simulink model "HQEV_MiL_20160830_integrate_r2017a"  (Simulink 8.9)
settings: Solver=FixedStepDiscrete  StartTime=0.0  StopTime=inf  FixedStep=0.01  RelTol=1e-3  EnableMultiTasking=on
PostLoadFcn:
  | , if any(exist('dsrtsu_mdlpostloadfcn', 'file') == [2, 3, 6]), try dsrtsu_mdlpostloadfcn('Execute', bdroot); catch fprintf('Error in PostLoadFcn (dsrtsu_mdlpostloadfcn) for model "%s":\n %s\n', bdroot, lasterr); end, end,
values from neighbouring files (symbols this model uses):
  Bat_C_Ah = 36    [parameter_V1.mat]
  Bat_ocv_xIndex = [5 10 20 30 40 50 60 70 80 90 95]    [parameter_V1.mat]
  Bat_ocv_z = [329 332 340 345 347 351 358 372 377 386 391]    [parameter_V1.mat]
  Bat_R_ohm_z = [4.41 3.46 1.57 1.07 0.76 0.63 0.55 0.44 0.41 0.4 0.4 3.14 ... (66 elements, 11x6)]    [parameter_V1.mat]
  Bat_SOC_Init = 90    [parameter_V1.mat]
  Env_hum_pct_Ambient = 30    [parameter_V1.mat]
  Env_Slope_deg = 0    [parameter_V1.mat]
  Env_Temp_degC_Ambient = 25    [parameter_V1.mat]
  Env_v_kmph_HWind = 0    [parameter_V1.mat]
  Reducer_F_i = 7.23    [parameter_V1.mat]
  Reducer_R_i = 7.23    [parameter_V1.mat]
  Veh =     [parameter_V1.mat]
  Veh_A_m2_Fr = 2.246    [parameter_V1.mat]
  Veh_F_Brake =     [parameter_V1.mat]
  Veh_fac_AirDrag = 0.326    [parameter_V1.mat]
  Veh_fac_WhDragFrict_0 = 0.011    [parameter_V1.mat]
  Veh_g_mps2_C = 9.81    [parameter_V1.mat]
  Veh_GainBrake =     [parameter_V1.mat]
  Veh_h_m_COGHigh = 0.5    [parameter_V1.mat]
  Veh_J_kgm2_Wh = 1.3635    [parameter_V1.mat]
  Veh_L_m_AxlBas = 2.63    [parameter_V1.mat]
  Veh_M_kg = 1427    [parameter_V1.mat]
  Veh_mu_Brake = 0.4    [parameter_V1.mat]
  Veh_mu_Tyre =     [parameter_V1.mat]
  Veh_num_FrictPair = 8    [parameter_V1.mat]
  Veh_pct_Brk = 70    [parameter_V1.mat]
  Veh_r_dyn =     [parameter_V1.mat]
  Veh_r_m_BrkDisk = 0.136    [parameter_V1.mat]
  Veh_rho_kgpm3_Air = 1.2258    [parameter_V1.mat]
undefined symbols (not defined in the file or in its folder): DiscIntNeverNeededParam, p_bool_False_M, p_bool_True_M
libraries: BaseOperationLib_Browser x38, simulink x8, DTQC_lib x1, ERR_lib x1, MQM_lib x1, PTCL_lib x1, PUD_lib x1, TQD_lib x1, TQR_lib x1, VMM_lib x1, ACCA_lib x1, BBCA_lib x1
(part 2 of 15)

== system HQEV_MiL_20160830_integrate_r2017a/MiL/Test_Integration/EGSM/EGSM ==
  In1 : Inport
  Bus Selector : BusSelector  OutputSignals=Drv.signal2.ParkButton (signal 11),Drv.signal2.SecurityButton (signal 12),Drv.signal2.EGSM_KnobPosition (signal 13),Drv.signal2.EGSM_ECOSButton (signal 14)
  Constant{,1..7} (8 alike) : Constant  Value=0
  Checksum_EGSM_1 : Outport
  EGSM_ParkButton : Outport  Port=2
  EGSM_SecurityButton : Outport  Port=3
  EGSM_KnobPosition : Outport  Port=4
  EGSMErrorStatus : Outport  Port=5
  EGSM_ECOSButton : Outport  Port=6
  LiveCounter_EGSM_1 : Outport  Port=7
  PowerSupplyStatus : Outport  Port=8
  EGSM_CANError : Outport  Port=9
  EGSM_LINError : Outport  Port=10
  EGSM_HallSensorError : Outport  Port=11
  EGSM_InternalError : Outport  Port=12
  wires:
  In1/1 -> Bus Selector/1
  Constant/1 -> Checksum_EGSM_1/1
  Constant1/1 -> EGSMErrorStatus/1
  Constant2/1 -> LiveCounter_EGSM_1/1
  Constant3/1 -> PowerSupplyStatus/1
  Constant4/1 -> EGSM_CANError/1
  Constant5/1 -> EGSM_LINError/1
  Constant6/1 -> EGSM_HallSensorError/1
  Constant7/1 -> EGSM_InternalError/1
  Bus Selector/1 -> EGSM_ParkButton/1  "<ParkButton (signal 11)>"
  Bus Selector/2 -> EGSM_SecurityButton/1  "<SecurityButton (signal 12)>"
  Bus Selector/3 -> EGSM_KnobPosition/1  "<EGSM_KnobPosition (signal 13)>"
  Bus Selector/4 -> EGSM_ECOSButton/1  "<EGSM_ECOSButton (signal 14)>"

== system HQEV_MiL_20160830_integrate_r2017a/MiL/Test_Integration/EPS/EPS ==
  Bus Creator : BusCreator  Inputs=2
  Subsystem2 : Subsystem
  EPS : Outport
  wires:
  Subsystem2/2(SteeringWheelAngleStatus) -> Bus Creator/2  "SteeringWheelAngleStatus"
  Subsystem2/1(EPSErrorStatus) -> Bus Creator/1  "EPSErrorStatus"
  Bus Creator/1 -> EPS/1

== system HQEV_MiL_20160830_integrate_r2017a/MiL/Test_Integration/ESP/Subsystem ==
  In1 : Inport
  ABS : Subsystem
  ASR : Subsystem
  ASR2 : Subsystem
  Bus Creator1 : BusCreator  Inputs=18
  Bus Creator2 : BusCreator  Inputs=6
  Bus Creator3 : BusCreator  Inputs=10
  Bus Creator4 : BusCreator  Inputs=4
  Bus Creator5 : BusCreator  Inputs=5
  Bus Creator6 : BusCreator  Inputs=6
  EPB : Subsystem
  YRS : Subsystem
  ESP : Outport
  wires:
  ABS/1(Checksum_ABS_1) -> Bus Creator1/1  "Checksum_ABS_1"
  ABS/2(WheelSpeed_FL) -> Bus Creator1/2  "WheelSpeed_FL"
  ABS/3(WheelSpeed_FR) -> Bus Creator1/3  "WheelSpeed_FR"
  ABS/4(ABS_VehicleSpeed) -> Bus Creator1/4  "ABS_VehicleSpeed"
  ABS/5(LiveCounter_ABS_1) -> Bus Creator1/5  "LiveCounter_ABS_1"
  ABS/6(Checksum_ABS_2) -> Bus Creator1/6  "Checksum_ABS_2"
  ABS/7(WheelSpeed_RL) -> Bus Creator1/7  "WheelSpeed_RL"
  ABS/8(WheelSpeed_RR) -> Bus Creator1/8  "WheelSpeed_RR"
  ABS/9(ABS_MasterCylinderPressure) -> Bus Creator1/9  "ABS_MasterCylinderPressure"
  ABS/10(LiveCounter_ABS_2) -> Bus Creator1/10  "LiveCounter_ABS_2"
  ABS/11(ABS_ErrorStatus) -> Bus Creator1/11  "ABS_ErrorStatus"
  ABS/12(ABS_Intervention) -> Bus Creator1/12  "ABS_Intervention"
  ABS/13(ASR_ErrorStatus) -> Bus Creator1/13  "ASR_ErrorStatus"
  ABS/14(ASR_Intervention) -> Bus Creator1/14  "ASR_Intervention"
  ABS/15(ESP_ErrorStatus) -> Bus Creator1/15  "ESP_ErrorStatus"
  ABS/16(ESP_Intervention) -> Bus Creator1/16  "ESP_Intervention"
  ABS/17(HHC_Status) -> Bus Creator1/17  "HHC_Status"
  ABS/18(HHC_Available) -> Bus Creator1/18  "HHC_Available"
  ASR/1(Checksum_ASR_1) -> Bus Creator2/1  "Checksum_ASR_1"
  ASR/2(ASR_TorqueReductionFast) -> Bus Creator2/2  "ASR_TorqueReductionFast"
  ASR/3(MSR_TorqueIncrease) -> Bus Creator2/3  "MSR_TorqueIncrease"
  ASR/4(LiveCounter_ASR_1) -> Bus Creator2/4  "LiveCounter_ASR_1"
  ASR/5(ASR_StatusTRFast) -> Bus Creator2/5  "ASR_StatusTRFast"
  ASR/6(MSR_StatusTI) -> Bus Creator2/6  "MSR_StatusTI"
  YRS/1(Checksum_YRS_1) -> Bus Creator3/1  "Checksum_YRS_1"
  YRS/2(AX1) -> Bus Creator3/2  "AX1"
  YRS/3(AY1) -> Bus Creator3/3  "AY1"
  YRS/4(LiveCounter_YRS_1) -> Bus Creator3/4  "LiveCounter_YRS_1"
  YRS/5(YRSStatus) -> Bus Creator3/5  "YRSStatus"
  YRS/6(YRSErrorStatus) -> Bus Creator3/6  "YRSErrorStatus"
  YRS/7(Checksum_YRS2) -> Bus Creator3/7  "Checksum_YRS2"
  YRS/8(AX1Offset) -> Bus Creator3/8  "AX1Offset"
  YRS/9(AY1Offset) -> Bus Creator3/9  "AY1Offset"
  YRS/10(LiveCounter_YRS2) -> Bus Creator3/10  "LiveCounter_YRS2"
  EPB/1(Checksum_EPB_1) -> Bus Creator4/1  "Checksum_EPB_1"
  EPB/2(LiveCounter_EPB_1) -> Bus Creator4/2  "LiveCounter_EPB_1"
  EPB/3(EPB_Status) -> Bus Creator4/3  "EPB_Status"
  EPB/4(EPB_ErrorStatus) -> Bus Creator4/4  "EPB_ErrorStatus"
  Bus Creator1/1 -> Bus Creator5/1  "ABS"
  Bus Creator2/1 -> Bus Creator5/2  "ASR"
  Bus Creator5/1 -> ESP/1
  In1/1 -> ABS/1(In1), ASR/1(In1), YRS/1(In1), EPB/1(In1), ASR2/1(In1)
  ASR2/5(ABS6RegenTrqReq) -> Bus Creator6/5  "ABS6RegenTrqReq"
  ASR2/4(ASR2StTIMSR2) -> Bus Creator6/4  "ASR2StTIMSR2"
  ASR2/6(ABS6StRegenTrqReq) -> Bus Creator6/6  "ABS6StRegenTrqReq"
  ASR2/3(ASR2StTRFastASR2) -> Bus Creator6/3  "ASR2StTRFastASR2"
  ASR2/2(ASR2TrqIncrsMSR2) -> Bus Creator6/2  "ASR2TrqIncrsMSR2"
  ASR2/1(ASR2TrqRdctFastASR2) -> Bus Creator6/1  "ASR2TrqRdctFastASR2"
  Bus Creator6/1 -> Bus Creator5/3  "ASR2"
  Bus Creator3/1 -> Bus Creator5/4  "YRS"
  Bus Creator4/1 -> Bus Creator5/5  "EPB"

== system HQEV_MiL_20160830_integrate_r2017a/MiL/Test_Integration/Enviroment/Environment ==
  note: mps=m/s
  note: pct=%
  Environment Air humidity : Constant  Value=Env_hum_pct_Ambient
  Environment Head Wind : Constant  Value=Env_v_kmph_HWind
  Environment Temp Ambient : Constant  Value=Env_Temp_degC_Ambient
  Slope : Constant  Value=Env_Slope_deg
  Slope_deg : Outport  Description=Current slope of the road [%]
  v_Hwind_mps : Outport  Description=Velocity of head wind [m/s]  Port=2
  Temp_Amb_degC : Outport  Description=Ambient temperature [degC]  Port=3
  Theta_Air_pct : Outport  Description=Ambient temperature [degC]  Port=4
  wires:
  Environment Temp Ambient/1 -> Temp_Amb_degC/1
  Environment Head Wind/1 -> v_Hwind_mps/1
  Environment Air humidity/1 -> Theta_Air_pct/1
  Slope/1 -> Slope_deg/1

== system HQEV_MiL_20160830_integrate_r2017a/MiL/Test_Integration/Epark/Subsystem ==
  In1 : Inport
  Bus Creator : BusCreator  Inputs=10
  Epark : Subsystem
  Rate Transition1 : RateTransition
  Rate Transition2 : RateTransition
  Rate Transition3 : RateTransition
  out : Outport
  wires:
  In1/1 -> Epark/1(In1)
  Epark/1(ePARK_MOTOR_OPEN_CKT) -> Bus Creator/1  "ePARK_MOTOR_OPEN_CKT"
  Epark/2(ePARK_MOTOR_JAMMED_PARK) -> Bus Creator/2  "ePARK_MOTOR_JAMMED_PARK"
  Epark/3(ePARK_MOTOR_JAMMED_UNPARK) -> Bus Creator/3  "ePARK_MOTOR_JAMMED_UNPARK"
  Epark/4(ePARK_MOTOR_JAMMED_MIDDL) -> Bus Creator/4  "ePARK_MOTOR_JAMMED_MIDDL"
  Epark/5(ePARK_HALL_SENSOR_INVALID) -> Bus Creator/5  "ePARK_HALL_SENSOR_INVALID"
  Epark/6(ePARK_LOST_COMM_VCU) -> Bus Creator/6  "ePARK_LOST_COMM_VCU"
  Epark/7(ePARK_CAN_ERR) -> Bus Creator/7  "ePARK_CAN_ERR"
  Epark/8(ParkLock) -> Rate Transition3/1  "ParkLock"
  Epark/9(ParkSensor) -> Rate Transition1/1  "ParkSensor"
  Epark/10(DriveSensor) -> Rate Transition2/1  "DriveSensor"
  Bus Creator/1 -> out/1
  Rate Transition1/1 -> Bus Creator/9  "ParkSensor"
  Rate Transition2/1 -> Bus Creator/10  "DriveSensor"
  Rate Transition3/1 -> Bus Creator/8  "ParkLock"
